simulink model "System_Model"  (R2021a)
settings: Solver=VariableStepAuto  StartTime=0.0  StopTime=10.0  RelTol=1e-3
settings Model: Creator=Hameed  LastModifiedBy=Hameed

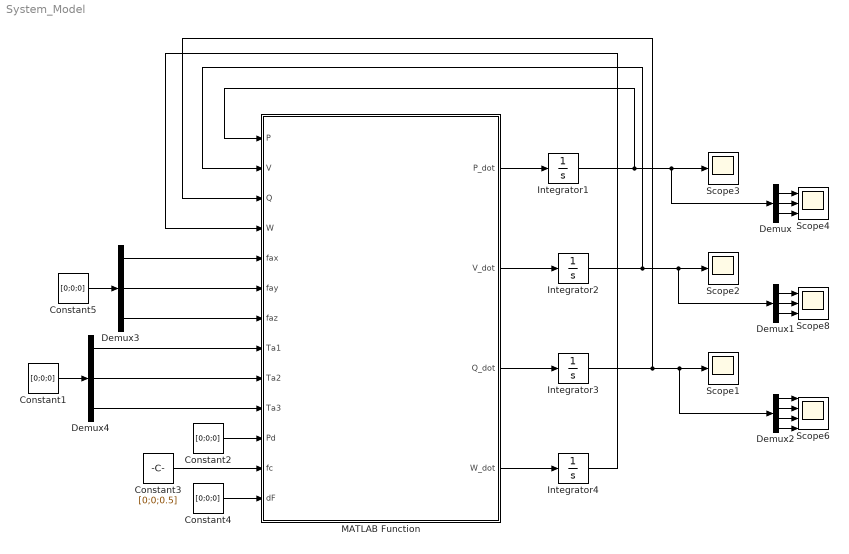
== system System_Model ==
  Constant{1..2,4..5} (4 alike) : Constant  Value=[0;0;0]  VectorParams1D=off
  Constant3 : Constant  Value=[0;0;0.5]  VectorParams1D=off
  Demux{,1,3..4} (4 alike) : Demux  Outputs=3
  Demux2 : Demux
  Integrator1 : Integrator  InitialCondition=[0;0;0]
  Integrator2 : Integrator  InitialCondition=[0;0;0]
  Integrator3 : Integrator  InitialCondition=[0;0;0;0]
  Integrator4 : Integrator  InitialCondition=[0;0;0]
  MATLAB Function : MATLAB Function  TreatAsAtomicUnit=on
  Scope1 : Scope
  Scope2 : Scope
  Scope3 : Scope
  Scope4 : Scope  NumInputPorts=3
  Scope6 : Scope  NumInputPorts=4
  Scope8 : Scope  NumInputPorts=3
  wires:
  Demux3/2 -> MATLAB Function/6(fay)
  Constant4/1 -> MATLAB Function/13(dF)
  Demux4/2 -> MATLAB Function/9(Ta2)
  Demux4/1 -> MATLAB Function/8(Ta1)
  Integrator4/1 -> MATLAB Function/4(W)
  Demux4/3 -> MATLAB Function/10(Ta3)
  Demux3/3 -> MATLAB Function/7(faz)
  Demux2/2 -> Scope6/2
  Demux2/1 -> Scope6/1
  Demux2/4 -> Scope6/4
  MATLAB Function/4(W_dot) -> Integrator4/1
  Demux1/1 -> Scope8/1
  Demux2/3 -> Scope6/3
  MATLAB Function/1(P_dot) -> Integrator1/1
  Demux1/2 -> Scope8/2
  Demux/3 -> Scope4/3
  Demux1/3 -> Scope8/3
  Demux3/1 -> MATLAB Function/5(fax)
  Integrator1/1 -> MATLAB Function/1(P), Scope3/1, Demux/1
  Demux/1 -> Scope4/1
  Constant3/1 -> MATLAB Function/12(fc)
  Demux/2 -> Scope4/2
  Integrator3/1 -> MATLAB Function/3(Q), Scope1/1, Demux2/1
  Constant2/1 -> MATLAB Function/11(Pd)
  MATLAB Function/3(Q_dot) -> Integrator3/1
  MATLAB Function/2(V_dot) -> Integrator2/1
  Integrator2/1 -> MATLAB Function/2(V), Scope2/1, Demux1/1
  Constant1/1 -> Demux4/1
  Constant5/1 -> Demux3/1

== matlab function System_Model/MATLAB Function ==
  data: P input; P_dot output; V input; Q input; W input; V_dot output; Q_dot output; W_dot output; fax input; fay input; faz input; Ta1 input; Ta2 input; Ta3 input; Pd input; fc input; dF input
function [P_dot,V_dot,Q_dot,W_dot]= fcn(P,V,Q,W,fax,fay,faz,Ta1,Ta2,Ta3,Pd,fc,dF)
clc
m=5;

% theta=Q(2);
% phi=Q(3);
% psi=Q(4);

% Rz=[cos(psi) sin(psi) 0;-sin(psi)) cos(psi) 0;0 0 1];
% Rx=[1 0 0;0 cos(theta) sin(theta);0 -sin(theta) cos(theta)];
% Ry=[cos(phi) 0 sin(phi);0 1 0;-sin(phi) 0 cos(phi)];

Rz=[cos(Q(4)) sin(Q(4)) 0;-sin(Q(4)) cos(Q(4)) 0;0 0 1];
Rx=[1 0 0;0 cos(Q(2)) sin(Q(2));0 -sin(Q(2)) cos(Q(2))];
Ry=[cos(Q(3)) 0 sin(Q(3));0 1 0;-sin(Q(3)) 0 cos(Q(3))];
Rb=Rz*Ry*Rx;
Rs=[1 0 0;0 0 -1;0 1 0 ];
%Rs=Rz*Rx*Ry;
%Rs=[1 0 0;0 -1 0;0 0 -1];
%lambda=L;
L=0;
%L=1;
Rd=[1 0 0;0 1 0;0 0 1-L];
SL=Rs*Rd*transpose(Rs);
%V=[Vx;Vy;Vz];
%Rb=Rz;
%Rb=[1 0 0;0 1 0;0 0 1];
%Rd=[1 0 0;0 1 0;0 0 1];
%fa=[fax;fay;faz];

P_dot=SL*V;
%rT=[rx;ry;rz];
%rT=P-Pd;
rT=[0.5;0;0];
%W=[Wx;Wy;Wz];

Q_dot=(1/2)*Q.*[0;W];

g=9.8;
%dF=[0;0;0.5];
dF=[0;0;0];
fc=[0;0;00];
%F=L*fc; as L=1
%F=fc;

% fax=fa(1);
% fay=fa(1);
% faz=fa(1);
% fa=[fax;fay;faz];
fa=[fax;fay;faz];
%fa=[fa(1);fa(2);fa(3)];
ab=(m^-1)*((Rb*fa)+(L*fc)+dF)+[0;0;g];

Ixx=1;
Iyy=1;
Izz=1;
J=[Ixx 0 0;0 Iyy 0;0 0 Izz];

%ta=[tx;ty;tz];
ta=[Ta1;Ta2;Ta3];

h=J*W;
rcom=[0;0;0];
%rcom=[0.05;0.05;0.05];
h1=transpose(Rb)*[0;0;m*g];
dT=[0;0;0];
%dT=[2;2;2];
h2=L*transpose(Rb)*fc;

W_dot=(inv(J))*(ta-cross(W,h)+cross(rcom,h1)+cross(rT,h2)+dT);

%ab=(m^-1)*((Rb*fa)+(L*fc)+dF)+[0;0;g];

V_dot=SL*((ab)+Rb*(cross(W_dot,rT)+(cross(W,cross(W,rT)))));
